simulink model "setpoint_quad1"  (R2016a)
settings: Solver=VariableStepAuto  StartTime=0.0  StopTime=inf  RelTol=1e-3
undefined symbols (not defined in the file): Pose
libraries: robotlib x3
settings Model: Creator=ttpl4  LastModifiedBy=UNIST
settings GRTTargetCC: GeneratePreprocessorConditionals=Use local settings

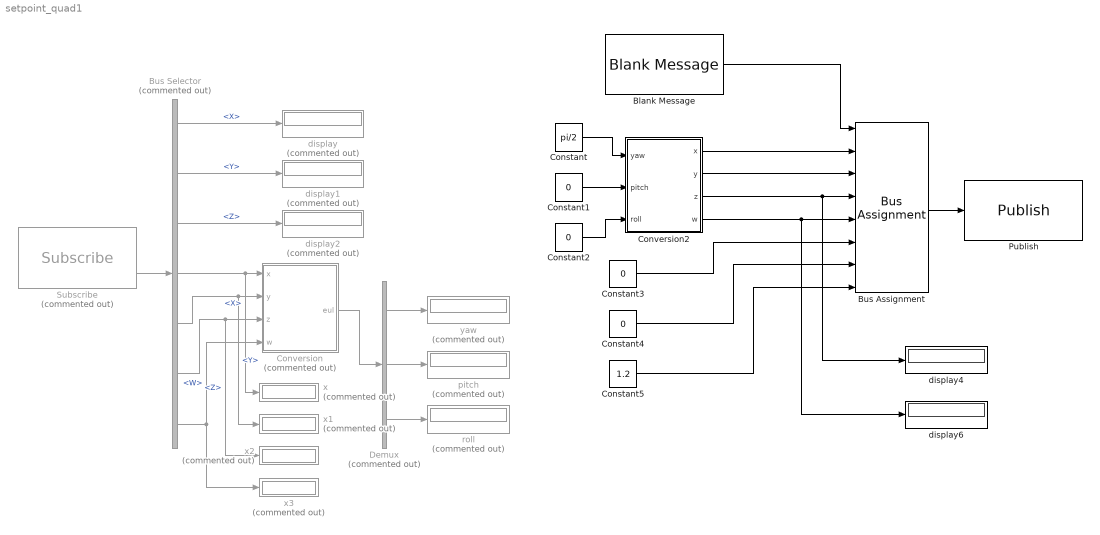
== system setpoint_quad1 ==
  Blank Message : robotlib/Blank Message  SourceLibraryInfo=This block requires Robotics System Toolbox  messageType=geometry_msgs/PoseStamped  SampleTime=-1
  Bus Assignment : BusAssignment  AssignedSignals=Pose.Orientation.X,Pose.Orientation.Y,Pose.Orientation.Z,Pose.Orientation.W,Pose.Position.X,Pose.Position.Y,Pose.Position.Z
  Bus Selector : BusSelector  Commented=on  OutputSignals=Pose.Position.X,Pose.Position.Y,Pose.Position.Z,Pose.Orientation.X,Pose.Orientation.Y,Pose.Orientation.Z,Pose.Orientation.W
  Constant : Constant  Value=pi/2
  Constant{1..4} (4 alike) : Constant  Value=0
  Constant5 : Constant  Value=1.2
  Conversion : MATLAB Function  Commented=on  TreatAsAtomicUnit=on
  Conversion2 : MATLAB Function  TreatAsAtomicUnit=on
  Demux : Demux  Commented=on  Outputs=3
  Publish : robotlib/Publish  SourceLibraryInfo=This block requires Robotics System Toolbox  topicSource=Select from ROS network  topic=/mavros/setpoint_position/local  messageType=geometry_msgs/PoseStamped  messageQueueLength=1
  Subscribe : robotlib/Subscribe  Commented=on  SourceLibraryInfo=This block requires Robotics System Toolbox  topicSource=Select from ROS network  topic=/mavros/local_position/pose  messageType=geometry_msgs/PoseStamped  sampleTime=-1  messageQueueLength=1
  display : Display  Commented=on
  display1 : Display  Commented=on
  display2 : Display  Commented=on
  display4 : Display
  display6 : Display
  pitch : Display  Commented=on
  roll : Display  Commented=on
  x{,1..3} (4 alike) : Display  Commented=on
  yaw : Display  Commented=on
  wires:
  Blank Message/1 -> Bus Assignment/1
  Bus Assignment/1 -> Publish/1
  Conversion2/4(w) -> Bus Assignment/5, display6/1
  Conversion2/3(z) -> display4/1, Bus Assignment/4
  Conversion2/2(y) -> Bus Assignment/3
  Conversion2/1(x) -> Bus Assignment/2
  Constant2/1 -> Conversion2/3(roll)
  Constant1/1 -> Conversion2/2(pitch)
  Constant/1 -> Conversion2/1(yaw)
  Constant3/1 -> Bus Assignment/6
  Constant4/1 -> Bus Assignment/7
  Constant5/1 -> Bus Assignment/8
  Bus Selector/1 -> display/1  "<X>"
  Bus Selector/2 -> display1/1  "<Y>"
  Bus Selector/3 -> display2/1  "<Z>"
  Bus Selector/4 -> x/1, Conversion/1(x)  "<X>"
  Bus Selector/5 -> x1/1, Conversion/2(y)  "<Y>"
  Bus Selector/6 -> x2/1, Conversion/3(z)  "<Z>"
  Bus Selector/7 -> Conversion/4(w), x3/1  "<W>"
  Conversion/1(eul) -> Demux/1
  Demux/1 -> yaw/1
  Demux/2 -> pitch/1
  Demux/3 -> roll/1
  Subscribe/2 -> Bus Selector/1

== matlab function setpoint_quad1/Conversion ==
  data: eul output; x input; y input; z input; w input
function eul  = quat2eul(x,y,z,w)
%#codegen

% Convert the quaternion to a yaw angle (zyx euler angle)
eul = quat2eul([w,x,y,z]);
% yaw = eul(1);

end

== matlab function setpoint_quad1/Conversion2 ==
  data: yaw input; pitch input; roll input; x output; y output; z output; w output
function [x,   y,   z,   w]   = eul2quat(yaw,pitch,roll)
%#codegen

% Convert the quaternion to a yaw angle (zyx euler angle)
q = eul2quat([yaw,pitch,roll]);
w=q(1);
x=q(2);
y=q(3);
z=q(4);
end
